simulink model "Uji_sisten"  (R2022b)
settings: Solver=VariableStepAuto  StartTime=0.0  StopTime=4000  RelTol=1e-3
libraries: slpidlib x2
settings Model: Creator=autom  LastModifiedBy=autom

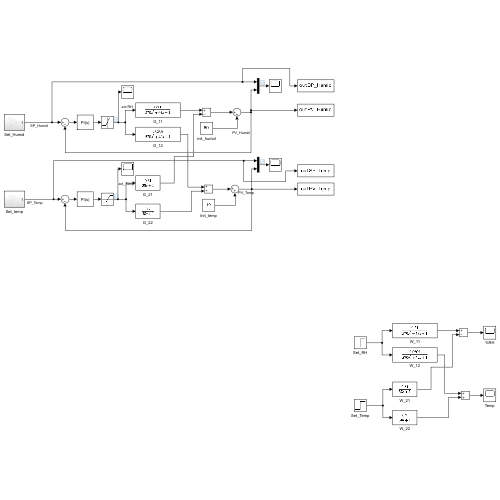
[thumbnail: Simulink's stored preview of the top-level diagram]
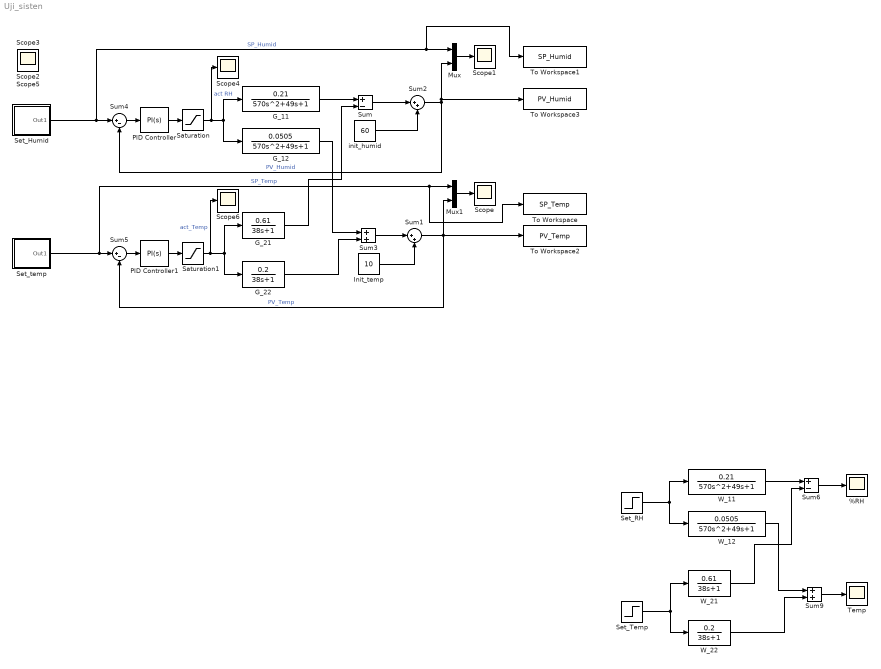
== system Uji_sisten ==
  %RH : Scope
  G_11 : TransferFcn  Numerator=[0.21]  Denominator=[570 49 1]
  G_12 : TransferFcn  Numerator=[0.0505]  Denominator=[570 49 1]
  G_21 : TransferFcn  Numerator=[0.61]  Denominator=[38 1]
  G_22 : TransferFcn  Numerator=[0.2]  Denominator=[38 1]
  Init_temp : Constant  Value=10
  Mux : Mux  Inputs=2
  Mux1 : Mux  Inputs=2
  PID Controller : slpidlib/PID Controller  Controller=PI  Form=Parallel  TimeDomain=Continuous-time  UseExternalTs=off  SampleTime=-1  IntegratorMethod=Forward Euler  FilterMethod=Forward Euler  ControllerParametersSource=internal  P=62.26  I=0.14  UseKiTs=off  D=0  N=100  UseFilter=on  TunerSelectOption=Transfer Function Based (PID Tuner App)  InitialConditionSource=internal  InitialConditionForIntegrator=0  InitialConditionForFilter=0  DifferentiatorICPrevScaledInput=0  ExternalReset=none  TrackingMode=off  Kt=1  LimitOutput=off  SatLimitsSource=internal  UpperSaturationLimit=inf  LowerSaturationLimit=-inf  LinearizeAsGain=on  AntiWindupMode=none  Kb=1  LimitIntegrator=off  UpperIntegratorSaturationLimit=inf  LowerIntegratorSaturationLimit=-inf  POutMin=[]  POutMax=[]  IOutMin=[]  IOutMax=[]  DOutMin=[]  DOutMax=[]  NOutMin=[]  NOutMax=[]  SumOutMin=[]  SumOutMax=[]  SaturationOutMin=[]  SaturationOutMax=[]  PParamMin=[]  PParamMax=[]  IParamMin=[]  IParamMax=[]  DParamMin=[]  DParamMax=[]  NParamMin=[]  NParamMax=[]  KbParamMin=[]  KbParamMax=[]  KtParamMin=[]  KtParamMax=[]  KbOutMin=[]  KbOutMax=[]  KtOutMin=[]  KtOutMax=[]  IntegratorOutMin=[]  IntegratorOutMax=[]  FilterOutMin=[]  FilterOutMax=[]  SumI1OutMin=[]  SumI1OutMax=[]  SumI2OutMin=[]  SumI2OutMax=[]  SumI3OutMin=[]  SumI3OutMax=[]  SumI4OutMin=[]  SumI4OutMax=[]  SumDOutMin=[]  SumDOutMax=[]  DifferentiatorOutMin=[]  DifferentiatorOutMax=[]  FilterDiffOutCoefMin=[]  FilterDiffOutCoefMax=[]  ReciprocalOutMin=[]  ReciprocalOutMax=[]  SumDenOutMin=[]  SumDenOutMax=[]  SumNumOutMin=[]  SumNumOutMax=[]  DivideOutMin=[]  DivideOutMax=[]  UdiffTsProdOutMin=[]  UdiffTsProdOutMax=[]  NTsProdOutMin=[]  NTsProdOutMax=[]  UintegralTsProdOutMin=[]  UintegralTsProdOutMax=[]  UngainTsProdOutMin=[]  UngainTsProdOutMax=[]  ClampingZeroOutDataTypeStr=Inherit: Inherit via back propagation  ClampingZeroOutMin=[]  ClampingZeroOutMax=[]  FilterDenConstantOutDataTypeStr=Inherit: Inherit via back propagation  FilterDenConstantOutMin=[]  FilterDenConstantOutMax=[]  PCopyOutDataTypeStr=Inherit: Inherit via back propagation  PCopyOutMin=[]  PCopyOutMax=[]  NCopyOutDataTypeStr=Inherit: Inherit via back propagation  NCopyOutMin=[]  NCopyOutMax=[]  IntegratorContinuousStateAttributes=''  IntegratorStateMustResolveToSignalObject=off  IntegratorRTWStateStorageClass=Auto  FilterContinuousStateAttributes=''  FilterStateMustResolveToSignalObject=off  FilterRTWStateStorageClass=Auto  ParallelPVariant=InternalParameters  IdealPVariant=Disabled  IVariant=InternalParameters  DVariant=Disabled  IntegratorVariant=Continuous  SatVariant=Disabled  AWVariant=Passthrough  PCopyVariant=Disabled  TRVariant=Disabled  FdbkBlocksVariant=Forward  IdealPFdbkVariant=Disabled  SatFdbkVariant=Disabled  DerivativeFilterVariant=Disabled  NVariant=Disabled  NCopyVariant=Disabled_SignalSpec  FilterICVariant=Disabled  IntegratorICVariant=InternalICs  ExternalResetVariant=Disabled  TRSumVariant=Passthrough  SumFdbkVariant=Disabled  SumVariant=Sum_PI  TsampFilterVariant=InternalTs  TsampNgainVariant=Passthrough  TsampIntegralVariant=Passthrough  ExternalSaturationOutDataTypeStr=Inherit: Same as second input
  PID Controller1 : slpidlib/PID Controller  Controller=PI  Form=Parallel  TimeDomain=Continuous-time  UseExternalTs=off  SampleTime=-1  IntegratorMethod=Forward Euler  FilterMethod=Forward Euler  ControllerParametersSource=internal  P=1.89  I=0.52  UseKiTs=off  D=0  N=100  UseFilter=on  TunerSelectOption=Transfer Function Based (PID Tuner App)  InitialConditionSource=internal  InitialConditionForIntegrator=0  InitialConditionForFilter=0  DifferentiatorICPrevScaledInput=0  ExternalReset=none  TrackingMode=off  Kt=1  LimitOutput=off  SatLimitsSource=internal  UpperSaturationLimit=inf  LowerSaturationLimit=-inf  LinearizeAsGain=on  AntiWindupMode=none  Kb=1  LimitIntegrator=off  UpperIntegratorSaturationLimit=inf  LowerIntegratorSaturationLimit=-inf  POutMin=[]  POutMax=[]  IOutMin=[]  IOutMax=[]  DOutMin=[]  DOutMax=[]  NOutMin=[]  NOutMax=[]  SumOutMin=[]  SumOutMax=[]  SaturationOutMin=[]  SaturationOutMax=[]  PParamMin=[]  PParamMax=[]  IParamMin=[]  IParamMax=[]  DParamMin=[]  DParamMax=[]  NParamMin=[]  NParamMax=[]  KbParamMin=[]  KbParamMax=[]  KtParamMin=[]  KtParamMax=[]  KbOutMin=[]  KbOutMax=[]  KtOutMin=[]  KtOutMax=[]  IntegratorOutMin=[]  IntegratorOutMax=[]  FilterOutMin=[]  FilterOutMax=[]  SumI1OutMin=[]  SumI1OutMax=[]  SumI2OutMin=[]  SumI2OutMax=[]  SumI3OutMin=[]  SumI3OutMax=[]  SumI4OutMin=[]  SumI4OutMax=[]  SumDOutMin=[]  SumDOutMax=[]  DifferentiatorOutMin=[]  DifferentiatorOutMax=[]  FilterDiffOutCoefMin=[]  FilterDiffOutCoefMax=[]  ReciprocalOutMin=[]  ReciprocalOutMax=[]  SumDenOutMin=[]  SumDenOutMax=[]  SumNumOutMin=[]  SumNumOutMax=[]  DivideOutMin=[]  DivideOutMax=[]  UdiffTsProdOutMin=[]  UdiffTsProdOutMax=[]  NTsProdOutMin=[]  NTsProdOutMax=[]  UintegralTsProdOutMin=[]  UintegralTsProdOutMax=[]  UngainTsProdOutMin=[]  UngainTsProdOutMax=[]  ClampingZeroOutDataTypeStr=Inherit: Inherit via back propagation  ClampingZeroOutMin=[]  ClampingZeroOutMax=[]  FilterDenConstantOutDataTypeStr=Inherit: Inherit via back propagation  FilterDenConstantOutMin=[]  FilterDenConstantOutMax=[]  PCopyOutDataTypeStr=Inherit: Inherit via back propagation  PCopyOutMin=[]  PCopyOutMax=[]  NCopyOutDataTypeStr=Inherit: Inherit via back propagation  NCopyOutMin=[]  NCopyOutMax=[]  IntegratorContinuousStateAttributes=''  IntegratorStateMustResolveToSignalObject=off  IntegratorRTWStateStorageClass=Auto  FilterContinuousStateAttributes=''  FilterStateMustResolveToSignalObject=off  FilterRTWStateStorageClass=Auto  ParallelPVariant=InternalParameters  IdealPVariant=Disabled  IVariant=InternalParameters  DVariant=Disabled  IntegratorVariant=Continuous  SatVariant=Disabled  AWVariant=Passthrough  PCopyVariant=Disabled  TRVariant=Disabled  FdbkBlocksVariant=Forward  IdealPFdbkVariant=Disabled  SatFdbkVariant=Disabled  DerivativeFilterVariant=Disabled  NVariant=Disabled  NCopyVariant=Disabled_SignalSpec  FilterICVariant=Disabled  IntegratorICVariant=InternalICs  ExternalResetVariant=Disabled  TRSumVariant=Passthrough  SumFdbkVariant=Disabled  SumVariant=Sum_PI  TsampFilterVariant=InternalTs  TsampNgainVariant=Passthrough  TsampIntegralVariant=Passthrough  ExternalSaturationOutDataTypeStr=Inherit: Same as second input
  Saturation : Saturate  UpperLimit=100  LowerLimit=0
  Saturation1 : Saturate  UpperLimit=100  LowerLimit=0
  Scope{,1..6} (7 alike) : Scope
  Set_Humid : Subsystem
  Set_RH : Step  SampleTime=0
  Set_Temp : Step  SampleTime=0
  Set_temp : Subsystem
  Sum : Sum  Inputs=+-
  Sum1 : Sum  Inputs=|++
  Sum2 : Sum  Inputs=|++
  Sum3 : Sum
  Sum4 : Sum  Inputs=|+-
  Sum5 : Sum  Inputs=|+-
  Sum6 : Sum  Inputs=+-
  Sum9 : Sum
  Temp : Scope
  To Workspace : ToWorkspace  VariableName=SP_Temp  SampleTime=1
  To Workspace1 : ToWorkspace  VariableName=SP_Humid  SampleTime=1
  To Workspace2 : ToWorkspace  VariableName=PV_Temp  SampleTime=1
  To Workspace3 : ToWorkspace  VariableName=PV_Humid  SaveFormat=Timeseries  SampleTime=1
  W_11 : TransferFcn  Numerator=[0.21]  Denominator=[570 49 1]
  W_12 : TransferFcn  Numerator=[0.0505]  Denominator=[570 49 1]
  W_21 : TransferFcn  Numerator=[0.61]  Denominator=[38 1]
  W_22 : TransferFcn  Numerator=[0.2]  Denominator=[38 1]
  init_humid : Constant  Value=60
  wires:
  Init_temp/1 -> Sum1/2
  init_humid/1 -> Sum2/2
  Sum1/1 -> To Workspace2/1, Sum5/2, Mux1/2  "PV_Temp"
  Sum3/1 -> Sum1/1
  Sum/1 -> Sum2/1
  G_11/1 -> Sum/1
  G_22/1 -> Sum3/2
  G_21/1 -> Sum/2
  G_12/1 -> Sum3/1
  Set_Humid/1(Out1) -> To Workspace1/1, Mux/1, Sum4/1  "SP_Humid"
  Sum2/1 -> To Workspace3/1, Mux/2, Sum4/2  "PV_Humid"
  Mux/1 -> Scope1/1
  Mux1/1 -> Scope/1
  Set_temp/1(Out1) -> Sum5/1, To Workspace/1, Mux1/1  "SP_Temp"
  Sum4/1 -> PID Controller/1
  PID Controller/1 -> Saturation/1
  Saturation/1 -> Scope4/1, G_12/1, G_11/1  "act RH"
  PID Controller1/1 -> Saturation1/1
  Sum5/1 -> PID Controller1/1
  Saturation1/1 -> Scope6/1, G_22/1, G_21/1  "act_Temp"
  Set_Temp/1 -> W_22/1, W_21/1
  Set_RH/1 -> W_12/1, W_11/1
  Sum6/1 -> %RH/1
  W_22/1 -> Sum9/2
  W_21/1 -> Sum6/2
  W_12/1 -> Sum9/1
  Sum9/1 -> Temp/1
  W_11/1 -> Sum6/1

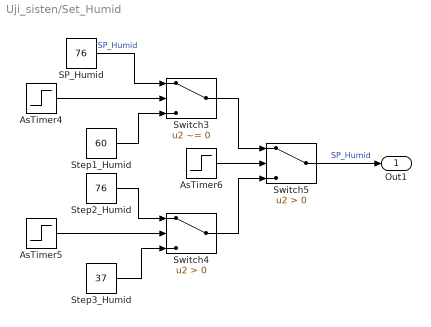
== system Uji_sisten/Set_Humid ==
  AsTimer4 : Step  Time=1000  Before=1  After=0  SampleTime=0
  AsTimer5 : Step  Time=3000  Before=1  After=0  SampleTime=0
  AsTimer6 : Step  Time=2000  Before=1  After=0  SampleTime=0
  SP_Humid : Constant  Value=76
  Step1_Humid : Constant  Value=60
  Step2_Humid : Constant  Value=76
  Step3_Humid : Constant  Value=37
  Switch3 : Switch  Criteria=u2 ~= 0  Threshold=1  SaturateOnIntegerOverflow=off  InputSameDT=off
  Switch4 : Switch  Criteria=u2 > Threshold  SaturateOnIntegerOverflow=off  InputSameDT=off
  Switch5 : Switch  Criteria=u2 > Threshold  SaturateOnIntegerOverflow=off  InputSameDT=off
  Out1 : Outport
  wires:
  SP_Humid/1 -> Switch3/1  "SP_Humid"
  Step3_Humid/1 -> Switch4/3
  Step1_Humid/1 -> Switch3/3
  AsTimer4/1 -> Switch3/2
  Switch3/1 -> Switch5/1
  AsTimer5/1 -> Switch4/2
  Step2_Humid/1 -> Switch4/1
  Switch4/1 -> Switch5/3
  AsTimer6/1 -> Switch5/2
  Switch5/1 -> Out1/1  "SP_Humid"

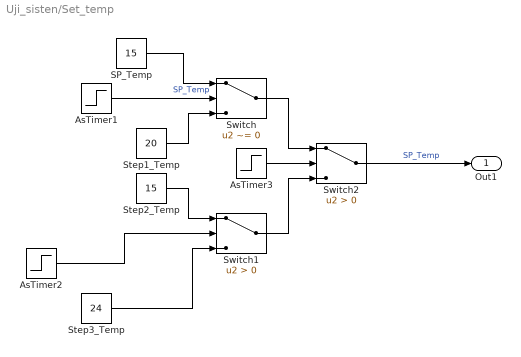
== system Uji_sisten/Set_temp ==
  AsTimer1 : Step  Time=1000  Before=1  After=0  SampleTime=0
  AsTimer2 : Step  Time=3000  Before=1  After=0  SampleTime=0
  AsTimer3 : Step  Time=2000  Before=1  After=0  SampleTime=0
  SP_Temp : Constant  Value=15
  Step1_Temp : Constant  Value=20
  Step2_Temp : Constant  Value=15
  Step3_Temp : Constant  Value=24
  Switch : Switch  Criteria=u2 ~= 0  Threshold=1  SaturateOnIntegerOverflow=off  InputSameDT=off
  Switch1 : Switch  Criteria=u2 > Threshold  SaturateOnIntegerOverflow=off  InputSameDT=off
  Switch2 : Switch  Criteria=u2 > Threshold  SaturateOnIntegerOverflow=off  InputSameDT=off
  Out1 : Outport
  wires:
  Switch/1 -> Switch2/1
  SP_Temp/1 -> Switch/1  "SP_Temp"
  Step3_Temp/1 -> Switch1/3
  Step1_Temp/1 -> Switch/3
  Step2_Temp/1 -> Switch1/1
  AsTimer3/1 -> Switch2/2
  AsTimer2/1 -> Switch1/2
  AsTimer1/1 -> Switch/2
  Switch1/1 -> Switch2/3
  Switch2/1 -> Out1/1  "SP_Temp"
